simulink model "tcp_simulink_example"  (R2023b)
settings: Solver=FixedStepAuto  StartTime=0.0  StopTime=inf  FixedStep=1e-3  RelTol=1e-3
libraries: slrealtimeiplib x6, slrealtimeutilitieslib x2, slrealtimeloglib x1, sldrtlib x1
settings Model: Creator=emu  LastModifiedBy=emu
settings SolverCC: ConcurrentTasks=on  PositivePriorityOrder=on
settings OptimizationCC: BlockReduction=off  OptimizeBlockIOStorage=off
settings DebuggingCC: TasksWithSamePriorityMsg=none
settings HardwareCC: ProdBitPerLong=64  ProdLongLongMode=on  ProdHWDeviceType=Intel->x86-64 (Linux 64)
settings RTWCC: Description=Simulink Real-Time  SystemTargetFile=slrealtime.tlc  TemplateMakefile=slrealtime_default_tmf  Toolchain=Simulink Real-Time Toolchain  BuildConfiguration=Faster Runs  CodeExecutionProfiling=on  TargetLang=C++

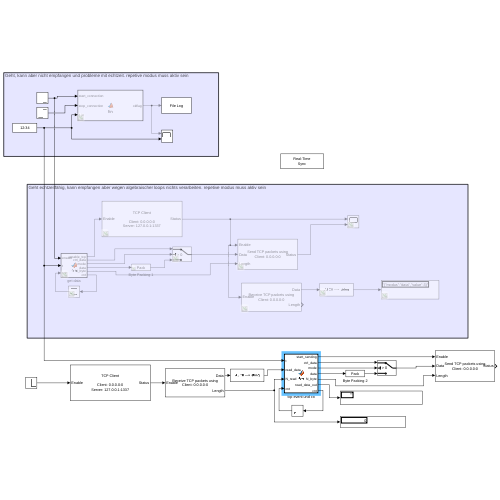
[thumbnail: Simulink's stored preview of the top-level diagram]
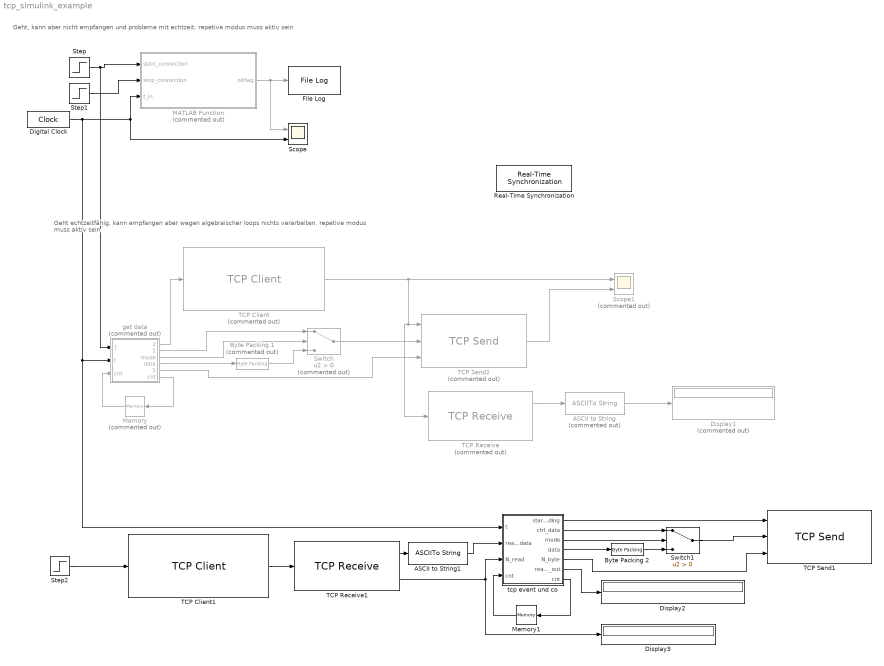
== system tcp_simulink_example ==
  note: Geht echtzeitfähig, kann empfangen aber wegen algebraischer loops nichts verarbeiten. repetive modus muss aktiv sein
  note: Geht, kann aber nicht empfangen und probleme mit echtzeit. repetive modus muss aktiv sein
  ASCII to String : ASCIIToString  Commented=on
  ASCII to String1 : ASCIIToString
  Byte Packing 1 : slrealtimeutilitieslib/Byte Packing  Commented=on  MaskPackedDataType=uint8  MaskUnpackedDataTypes={'double'}  MaskAlignment=1
  Byte Packing 2 : slrealtimeutilitieslib/Byte Packing  MaskPackedDataType=uint8  MaskUnpackedDataTypes={'double'}  MaskAlignment=1
  Digital Clock : DigitalClock  SampleTime=0.1
  Display1 : Display  Commented=on
  Display2 : Display
  Display3 : Display
  File Log : slrealtimeloglib/File Log  decimation=1  inputProcessing=Elements as channels (sample based)
  MATLAB Function : MATLAB Function  Commented=on  TreatAsAtomicUnit=on
  Memory : Memory  Commented=on  InheritSampleTime=on
  Memory1 : Memory  InheritSampleTime=on
  Real-Time Synchronization : sldrtlib/Real-Time Synchronization  SampleTime=0.1  MaxMissedTicks=10  ShowMissedTicks=off  YieldWhenWaiting=off
  Scope : Scope  NumInputPorts=2
  Scope1 : Scope  Commented=on  NumInputPorts=2
  Step : Step  Before=1  After=0  SampleTime=0.1
  Step1 : Step  SampleTime=0.1
  Step2 : Step  Time=100  Before=1  After=0  SampleTime=0.1
  Switch : Switch  Commented=on  Criteria=u2 > Threshold  SaturateOnIntegerOverflow=off  InputSameDT=off
  Switch1 : Switch  Criteria=u2 > Threshold  SaturateOnIntegerOverflow=off  InputSameDT=off
  TCP Client : slrealtimeiplib/TCP Client  Priority=-1  Commented=on  useHostTargetConn=off  remoteAddress=127.0.0.1  remotePort=1337
  TCP Client1 : slrealtimeiplib/TCP Client  Priority=-1  useHostTargetConn=off  remoteAddress=127.0.0.1  remotePort=1337
  TCP Receive : slrealtimeiplib/TCP Receive  Commented=on  socketAddPortVal=Client: 0.0.0.0:0  rcvWidth=26  sampleTime=-1
  TCP Receive1 : slrealtimeiplib/TCP Receive  socketAddPortVal=Client: 0.0.0.0:0  rcvWidth=26  sampleTime=-1
  TCP Send1 : slrealtimeiplib/TCP Send  socketAddPortVal=Client: 0.0.0.0:0  sampleTime=-1
  TCP Send2 : slrealtimeiplib/TCP Send  Commented=on  socketAddPortVal=Client: 0.0.0.0:0  sampleTime=-1
  get data : MATLAB Function  Commented=on  TreatAsAtomicUnit=on
  tcp event und co : MATLAB Function  TreatAsAtomicUnit=on
  wires:
  Step/1 -> MATLAB Function/1(start_connection), get data/1(enable)
  Step1/1 -> MATLAB Function/2(stop_connection)
  Digital Clock/1 -> tcp event und co/1(t), get data/2(t), Scope/2, MATLAB Function/3(t_in)
  MATLAB Function/1(okflag) -> Scope/1, File Log/1
  TCP Client/1 -> Scope1/1, TCP Receive/1, TCP Send2/1
  get data/5(N_byte) -> TCP Send2/3
  TCP Send2/1 -> Scope1/2
  get data/4(data) -> Byte Packing 1/1
  get data/3(mode) -> Switch/2
  get data/2(ctrl_data) -> Switch/1
  Byte Packing 1/1 -> Switch/3
  Switch/1 -> TCP Send2/2
  Memory/1 -> get data/3("cnt ")
  get data/6(cnt) -> Memory/1
  TCP Receive/1 -> ASCII to String/1
  ASCII to String/1 -> Display1/1
  get data/1(enable_tcp) -> TCP Client/1
  TCP Client1/1 -> TCP Receive1/1
  Step2/1 -> TCP Client1/1
  tcp event und co/1(start_sending) -> TCP Send1/1
  tcp event und co/7(cnt) -> Memory1/1
  Memory1/1 -> tcp event und co/4("cnt ")
  Byte Packing 2/1 -> Switch1/3
  tcp event und co/2(ctrl_data) -> Switch1/1
  tcp event und co/4(data) -> Byte Packing 2/1
  tcp event und co/3(mode) -> Switch1/2
  tcp event und co/5(N_byte) -> TCP Send1/3
  Switch1/1 -> TCP Send1/2
  TCP Receive1/1 -> ASCII to String1/1
  ASCII to String1/1 -> tcp event und co/2(read_data)
  TCP Receive1/2 -> Display3/1, tcp event und co/3(N_read)
  tcp event und co/6(read_data_out) -> Display2/1

== matlab function tcp_simulink_example/get data ==
  settings: updateMethod=DISCRETE  sampleTime=0.1
  data: enable_tcp output; ctrl_data output; mode output; enable input; data output; N_byte output; t input; cnt input; cnt output
function [enable_tcp, ctrl_data, mode, data, N_byte, cnt] = fcn(enable, t, cnt)

N_data=5000; %float64 daten: 8byte
N_byte = N_data*8;
ctrl_data=uint8('0');
data=zeros(1,N_data);
mode=1;
enable_tcp=0;

if(cnt==0 && enable == 1)
    enable_tcp=1;
    mode = 1;
    ctrl_data=uint8('0'); %send 0: start write
    N_byte=1; % NUR 1 BYTE
    cnt=1;
    %pause(0.01);
elseif(cnt==1)
    mode = -1;
    i_arr=linspace(0,1,N_data);
    data=cos(10*pi*i_arr*t) + 2.5*cos(2*pi*i_arr);
    cnt=2;
    enable_tcp=1;
elseif(cnt==2)
    mode = -1;
    i_arr=linspace(0,1,N_data);
    data=t+2.5*sin(2*pi*i_arr);
    cnt=0;
    enable_tcp=1;
elseif(cnt==3 || enable == 0)
    enable_tcp=0;
end

== matlab function tcp_simulink_example/MATLAB Function ==
  settings: updateMethod=DISCRETE  sampleTime=0.1
  data: start_connection input; okflag output; stop_connection input; t_in input
function okflag = fcn(start_connection, stop_connection, t_in)

    persistent started;
    persistent tcp_obj;
    persistent i;
    coder.extrinsic("tcpclient");
    coder.extrinsic("write");
    coder.extrinsic("configureCallback");


    if(isempty(started))
        started = 0;
        tcp_obj = tcpclient("127.0.0.1",1337);
        i=0;
    end

    %pause(0.1)
    
    if(started == 0 && start_connection == 1)
        i=i+1;
        started=1;
        N=5000;
        i_arr=linspace(0,1,N);
        data=2.5*cos(2*pi*i_arr);%+0.1*rand(1,5000);
    
        write(tcp_obj,'0'); %tcp client sagen, dass daten kommen
        write(tcp_obj,t_in-1+data);
        write(tcp_obj,data*2);
        %configureCallback(tcp_obj,"byte",26,@send_data);
    end
    
    if(stop_connection == 1)
        clear tcp_obj;
        started=0;
        %echotcpip("off");
    end
    %write(t,data);
    %write(t,data*10);
    
    %pause(1)
    %clear t
    %echotcpip("off")
    
    
    okflag=0;
    
    function send_data(t, event)
        fprintf("empfangen: %s\n", t.read())
        fprintf("send data\n")
        N=5000;
        i_arr=linspace(0,1,N);
        data=2.5*cos(2*pi*i_arr)+0.1*rand(1,5000);
    
        write(t,'0'); %tcp client sagen, dass daten kommen
        write(t,data);
        write(t,data*10);
    end
end

== matlab function tcp_simulink_example/tcp event und co ==
  settings: updateMethod=DISCRETE  sampleTime=0.1
  data: start_sending output; ctrl_data output; mode output; data output; N_byte output; read_data_out output; t input; read_data input; N_read input; cnt input; cnt output
function [start_sending, ctrl_data, mode, data, N_byte, read_data_out, cnt] = fcn(t, read_data, N_read, cnt)

N_data=5000; %float64 daten: 8byte
N_byte = N_data*8;
ctrl_data=uint8('0');
data=zeros(1,N_data);
mode=1;
start_sending=0;
read_data_out = read_data;

if(cnt==0) % read data
    if(N_read > 0)
        cnt=1; % start sending
    end
elseif(cnt==1)
    start_sending=1;
    mode = 1;
    ctrl_data=uint8('0'); %send 0: start write
    N_byte=1; % NUR 1 BYTE
    cnt=2;
    %pause(0.01);
elseif(cnt==2)
    mode = -1;
    i_arr=linspace(0,1,N_data);
    data=cos(10*pi*i_arr*t) + 2.5*cos(2*pi*i_arr);
    cnt=3;
    start_sending=1;
elseif(cnt==3)
    mode = -1;
    i_arr=linspace(0,1,N_data);
    data=t+2.5*sin(2*pi*i_arr);
    cnt=0;
    start_sending=1;
    read_data_out = "";
end
